simulink model "FunctionalArchitecture"  (R2022b)
settings: Solver=VariableStepAuto  StartTime=0.0  StopTime=10.0  RelTol=1e-3
undefined symbols (not defined in the file): Camera_data, Lidar, Posiont, Position, SpeedVacuum
settings Model: Creator=carol  LastModifiedBy=carol
settings OptimizationCC: ReuseModelBlockBuffer=on

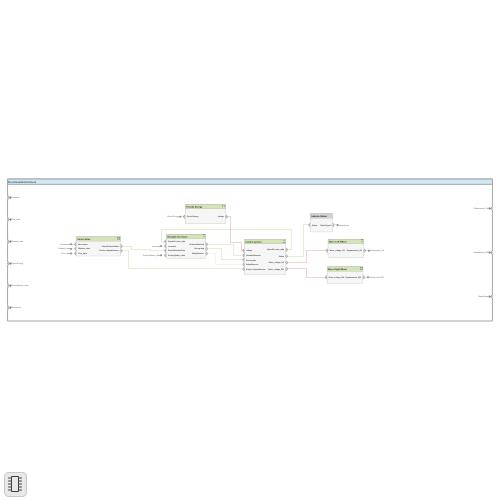
[thumbnail: Simulink's stored preview of the top-level diagram]
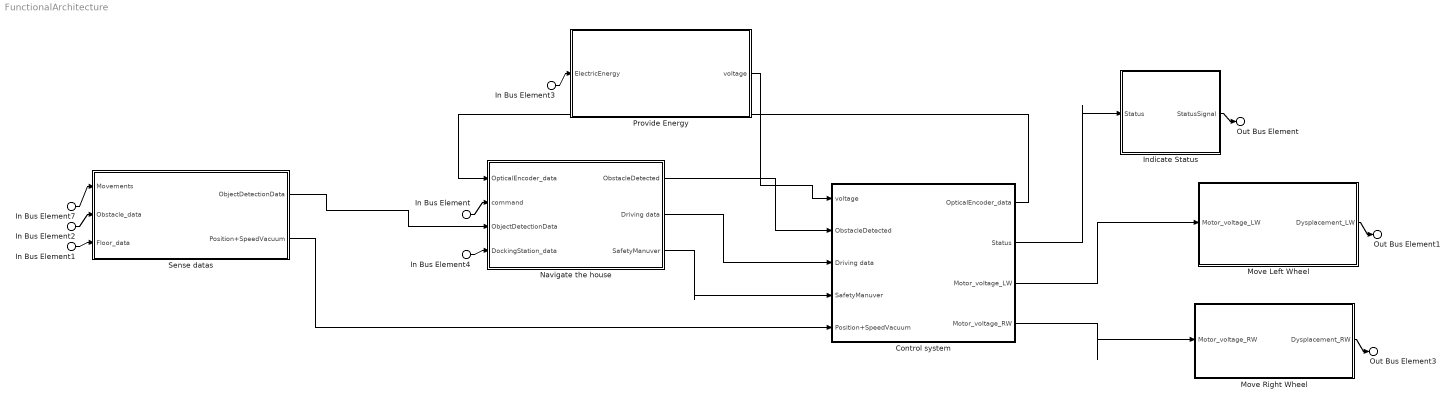
== system FunctionalArchitecture ==
  In Bus Element : Inport  PortName=command
  In Bus Element1 : Inport  Port=2  PortName=Floor_data
  In Bus Element2 : Inport  Port=3  PortName=Obstacle_data
  In Bus Element3 : Inport  Port=4  PortName=ElectricEnergy
  In Bus Element4 : Inport  Port=5  PortName=DockingStation_data
  In Bus Element7 : Inport  Port=6  PortName=Movements
  Control system : Subsystem
      settings: PortSchema="{\"entries\":[{\"content\":{\"headerSize\":26,\"margin\":15,\"minimumSpacing\":25,\"sides\":[{\"content\":{\"connectorIds\":[\"In1\",\"In2\",\"In4\",\"In3\",\"In5\"]},\"type\":\"ConnectorPlacement.EquallySpacedRectSide\",\"uuid\":\"6ae6270c-bff4-4a0d-8fba-8fdec87b0a05\"},{\"content\":{\"connectorIds\":[\"Out1\",\"Out2\",\"Out3\",\"Out4\"],\"side\":\"RIGHT\"},\"type\":\"ConnectorPlacement.EquallySpacedRectSide\",\"uuid\":\"f3a0045b-bb3b-40f9-afd5-e1537ff3eeca\"},{\"content\":{\"side\":\"TOP\"},\"type\":\"ConnectorPlacement.EquallySpacedRectSide\",\"uuid\":\"e89a58f2-90b0-468c-bb6a-95617af68e24\"}]},\"type\":\"ConnectorPlacement.EquallySpacedConnector\",\"uuid\":\"066eb43c-7b96-4660-9f29-628dd77a5b3b\"}],\"packageUris\":[\"http://schema.mathworks.com/mf0/Connector/R2020b\"],\"version\":\"1.0\"}"
  Indicate Status : Subsystem
      settings: PortSchema="{\"entries\":[{\"content\":{\"headerSize\":26,\"margin\":15,\"minimumSpacing\":25,\"sides\":[{\"content\":{\"connectorIds\":[\"In1\"]},\"type\":\"ConnectorPlacement.EquallySpacedRectSide\",\"uuid\":\"9cca9539-0a36-4124-b22c-ee31f3591a67\"},{\"content\":{\"connectorIds\":[\"Out1\"],\"side\":\"RIGHT\"},\"type\":\"ConnectorPlacement.EquallySpacedRectSide\",\"uuid\":\"eebe1ec1-c849-468b-8863-53f0cc841d23\"},{\"content\":{\"side\":\"TOP\"},\"type\":\"ConnectorPlacement.EquallySpacedRectSide\",\"uuid\":\"8f1c4dda-9d7f-4fb5-99d0-4e96ed432329\"}]},\"type\":\"ConnectorPlacement.EquallySpacedConnector\",\"uuid\":\"f7d57f3a-667c-4dfa-8f30-8433699dfbc6\"}],\"packageUris\":[\"http://schema.mathworks.com/mf0/Connector/R2020b\"],\"version\":\"1.0\"}"
  Move Left Wheel : Subsystem
      settings: PortSchema="{\"entries\":[{\"content\":{\"headerSize\":26,\"margin\":15,\"minimumSpacing\":25,\"sides\":[{\"content\":{\"connectorIds\":[\"In1\"]},\"type\":\"ConnectorPlacement.EquallySpacedRectSide\",\"uuid\":\"6ae6270c-bff4-4a0d-8fba-8fdec87b0a05\"},{\"content\":{\"connectorIds\":[\"Out1\"],\"side\":\"RIGHT\"},\"type\":\"ConnectorPlacement.EquallySpacedRectSide\",\"uuid\":\"f3a0045b-bb3b-40f9-afd5-e1537ff3eeca\"},{\"content\":{\"side\":\"TOP\"},\"type\":\"ConnectorPlacement.EquallySpacedRectSide\",\"uuid\":\"e89a58f2-90b0-468c-bb6a-95617af68e24\"}]},\"type\":\"ConnectorPlacement.EquallySpacedConnector\",\"uuid\":\"066eb43c-7b96-4660-9f29-628dd77a5b3b\"}],\"packageUris\":[\"http://schema.mathworks.com/mf0/Connector/R2020b\"],\"version\":\"1.0\"}"
  Move Right Wheel : Subsystem
      settings: PortSchema="{\"entries\":[{\"content\":{\"headerSize\":26,\"margin\":15,\"minimumSpacing\":25,\"sides\":[{\"content\":{\"connectorIds\":[\"In1\"]},\"type\":\"ConnectorPlacement.EquallySpacedRectSide\",\"uuid\":\"6ae6270c-bff4-4a0d-8fba-8fdec87b0a05\"},{\"content\":{\"connectorIds\":[\"Out1\"],\"side\":\"RIGHT\"},\"type\":\"ConnectorPlacement.EquallySpacedRectSide\",\"uuid\":\"f3a0045b-bb3b-40f9-afd5-e1537ff3eeca\"},{\"content\":{\"side\":\"TOP\"},\"type\":\"ConnectorPlacement.EquallySpacedRectSide\",\"uuid\":\"e89a58f2-90b0-468c-bb6a-95617af68e24\"}]},\"type\":\"ConnectorPlacement.EquallySpacedConnector\",\"uuid\":\"066eb43c-7b96-4660-9f29-628dd77a5b3b\"}],\"packageUris\":[\"http://schema.mathworks.com/mf0/Connector/R2020b\"],\"version\":\"1.0\"}"
  Navigate the house : Subsystem
      settings: PortSchema="{\"entries\":[{\"content\":{\"headerSize\":26,\"margin\":15,\"minimumSpacing\":25,\"sides\":[{\"content\":{\"connectorIds\":[\"In1\",\"In2\",\"In3\",\"In4\"]},\"type\":\"ConnectorPlacement.EquallySpacedRectSide\",\"uuid\":\"9cca9539-0a36-4124-b22c-ee31f3591a67\"},{\"content\":{\"connectorIds\":[\"Out1\",\"Out3\",\"Out2\"],\"side\":\"RIGHT\"},\"type\":\"ConnectorPlacement.EquallySpacedRectSide\",\"uuid\":\"eebe1ec1-c849-468b-8863-53f0cc841d23\"},{\"content\":{\"side\":\"TOP\"},\"type\":\"ConnectorPlacement.EquallySpacedRectSide\",\"uuid\":\"8f1c4dda-9d7f-4fb5-99d0-4e96ed432329\"}]},\"type\":\"ConnectorPlacement.EquallySpacedConnector\",\"uuid\":\"f7d57f3a-667c-4dfa-8f30-8433699dfbc6\"}],\"packageUris\":[\"http://schema.mathworks.com/mf0/Connector/R2020b\"],\"version\":\"1.0\"}"
  Provide Energy : Subsystem
      settings: PortSchema="{\"entries\":[{\"content\":{\"headerSize\":26,\"margin\":15,\"minimumSpacing\":25,\"sides\":[{\"content\":{\"connectorIds\":[\"In1\"]},\"type\":\"ConnectorPlacement.EquallySpacedRectSide\",\"uuid\":\"6ae6270c-bff4-4a0d-8fba-8fdec87b0a05\"},{\"content\":{\"connectorIds\":[\"Out1\"],\"side\":\"RIGHT\"},\"type\":\"ConnectorPlacement.EquallySpacedRectSide\",\"uuid\":\"f3a0045b-bb3b-40f9-afd5-e1537ff3eeca\"},{\"content\":{\"side\":\"TOP\"},\"type\":\"ConnectorPlacement.EquallySpacedRectSide\",\"uuid\":\"e89a58f2-90b0-468c-bb6a-95617af68e24\"}]},\"type\":\"ConnectorPlacement.EquallySpacedConnector\",\"uuid\":\"066eb43c-7b96-4660-9f29-628dd77a5b3b\"}],\"packageUris\":[\"http://schema.mathworks.com/mf0/Connector/R2020b\"],\"version\":\"1.0\"}"
  Sense datas : Subsystem
      settings: PortSchema="{\"entries\":[{\"content\":{\"headerSize\":26,\"margin\":15,\"minimumSpacing\":25,\"sides\":[{\"content\":{\"connectorIds\":[\"In1\",\"In2\",\"In3\"]},\"type\":\"ConnectorPlacement.EquallySpacedRectSide\",\"uuid\":\"6ae6270c-bff4-4a0d-8fba-8fdec87b0a05\"},{\"content\":{\"connectorIds\":[\"Out2\",\"Out1\"],\"side\":\"RIGHT\"},\"type\":\"ConnectorPlacement.EquallySpacedRectSide\",\"uuid\":\"f3a0045b-bb3b-40f9-afd5-e1537ff3eeca\"},{\"content\":{\"side\":\"TOP\"},\"type\":\"ConnectorPlacement.EquallySpacedRectSide\",\"uuid\":\"e89a58f2-90b0-468c-bb6a-95617af68e24\"}]},\"type\":\"ConnectorPlacement.EquallySpacedConnector\",\"uuid\":\"066eb43c-7b96-4660-9f29-628dd77a5b3b\"}],\"packageUris\":[\"http://schema.mathworks.com/mf0/Connector/R2020b\"],\"version\":\"1.0\"}"
  Out Bus Element1 : Outport  PortName=Displacement_LW
  Out Bus Element3 : Outport  Port=2  PortName=Displacement_RW
  Out Bus Element : Outport  Port=3  PortName=StatusSignal
  wires:
  Navigate the house/3(Driving data) -> Control system/4(Driving data)
  Provide Energy/1(voltage) -> Control system/1(voltage)
  In Bus Element3/1 -> Provide Energy/1(ElectricEnergy)
  Control system/3(Motor_voltage_LW) -> Move Left Wheel/1(Motor_voltage_LW)
  Control system/4(Motor_voltage_RW) -> Move Right Wheel/1(Motor_voltage_RW)
  Move Left Wheel/1(Dysplacement_LW) -> Out Bus Element1/1
  Move Right Wheel/1(Dysplacement_RW) -> Out Bus Element3/1
  In Bus Element7/1 -> Sense datas/1(Movements)
  In Bus Element2/1 -> Sense datas/2(Obstacle_data)
  In Bus Element1/1 -> Sense datas/3(Floor_data)
  Sense datas/2(ObjectDetectionData) -> Navigate the house/3(ObjectDetectionData)
  Sense datas/1(Position+SpeedVacuum) -> Control system/5(Position+SpeedVacuum)
  In Bus Element/1 -> Navigate the house/2(command)
  In Bus Element4/1 -> Navigate the house/4(DockingStation_data)
  Control system/1(OpticalEncoder_data) -> Navigate the house/1(OpticalEncoder_data)
  Indicate Status/1(StatusSignal) -> Out Bus Element/1
  Control system/2(Status) -> Indicate Status/1(Status)
  Navigate the house/1(ObstacleDetected) -> Control system/2(ObstacleDetected)
  Navigate the house/2(SafetyManuver) -> Control system/3(SafetyManuver)

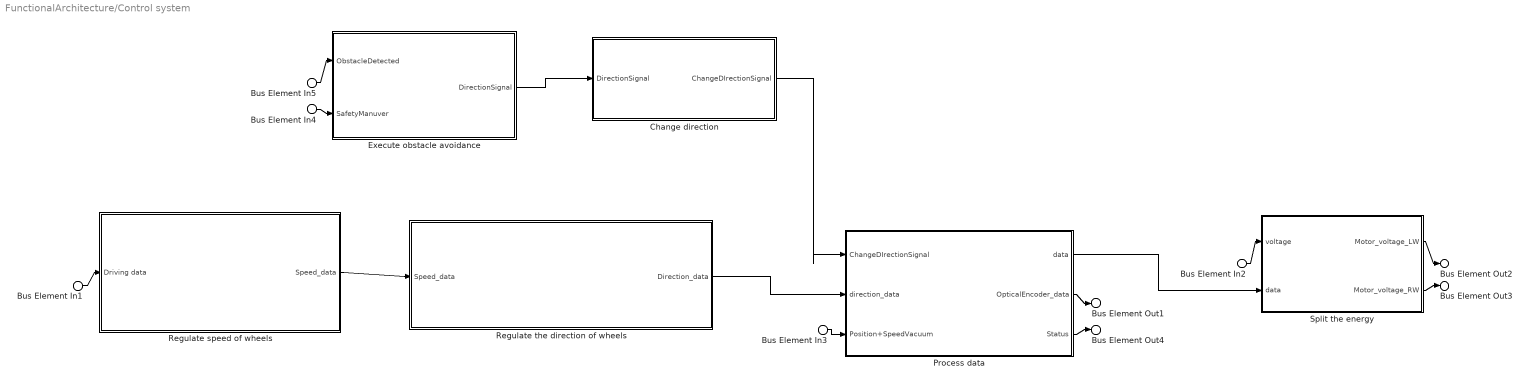
== system FunctionalArchitecture/Control system ==
  Bus Element In2 : Inport  PortName=voltage
  Bus Element In5 : Inport  Port=2  PortName=ObstacleDetected
  Bus Element In4 : Inport  Port=3  PortName=SafetyManuver
  Bus Element In1 : Inport  Port=4  PortName=Driving data
  Bus Element In3 : Inport  Port=5  PortName=Position+SpeedVacuum
  Change direction : Subsystem
      settings: PortSchema="{\"entries\":[{\"content\":{\"headerSize\":26,\"margin\":15,\"minimumSpacing\":25,\"sides\":[{\"content\":{\"connectorIds\":[\"In1\"]},\"type\":\"ConnectorPlacement.EquallySpacedRectSide\",\"uuid\":\"9cca9539-0a36-4124-b22c-ee31f3591a67\"},{\"content\":{\"connectorIds\":[\"Out1\"],\"side\":\"RIGHT\"},\"type\":\"ConnectorPlacement.EquallySpacedRectSide\",\"uuid\":\"eebe1ec1-c849-468b-8863-53f0cc841d23\"},{\"content\":{\"side\":\"TOP\"},\"type\":\"ConnectorPlacement.EquallySpacedRectSide\",\"uuid\":\"8f1c4dda-9d7f-4fb5-99d0-4e96ed432329\"}]},\"type\":\"ConnectorPlacement.EquallySpacedConnector\",\"uuid\":\"f7d57f3a-667c-4dfa-8f30-8433699dfbc6\"}],\"packageUris\":[\"http://schema.mathworks.com/mf0/Connector/R2020b\"],\"version\":\"1.0\"}"
  Execute obstacle avoidance : Subsystem
      settings: PortSchema="{\"entries\":[{\"content\":{\"headerSize\":26,\"margin\":15,\"minimumSpacing\":25,\"sides\":[{\"content\":{\"connectorIds\":[\"In1\",\"In2\"]},\"type\":\"ConnectorPlacement.EquallySpacedRectSide\",\"uuid\":\"9cca9539-0a36-4124-b22c-ee31f3591a67\"},{\"content\":{\"connectorIds\":[\"Out1\"],\"side\":\"RIGHT\"},\"type\":\"ConnectorPlacement.EquallySpacedRectSide\",\"uuid\":\"eebe1ec1-c849-468b-8863-53f0cc841d23\"},{\"content\":{\"side\":\"TOP\"},\"type\":\"ConnectorPlacement.EquallySpacedRectSide\",\"uuid\":\"8f1c4dda-9d7f-4fb5-99d0-4e96ed432329\"}]},\"type\":\"ConnectorPlacement.EquallySpacedConnector\",\"uuid\":\"f7d57f3a-667c-4dfa-8f30-8433699dfbc6\"}],\"packageUris\":[\"http://schema.mathworks.com/mf0/Connector/R2020b\"],\"version\":\"1.0\"}"
  Process data : Subsystem
      settings: PortSchema="{\"entries\":[{\"content\":{\"headerSize\":26,\"margin\":15,\"minimumSpacing\":25,\"sides\":[{\"content\":{\"connectorIds\":[\"In1\",\"In2\",\"In3\"]},\"type\":\"ConnectorPlacement.EquallySpacedRectSide\",\"uuid\":\"c0b5e0bb-d2bf-4d40-b1ad-0d63f5f2311e\"},{\"content\":{\"connectorIds\":[\"Out1\",\"Out2\",\"Out3\"],\"side\":\"RIGHT\"},\"type\":\"ConnectorPlacement.EquallySpacedRectSide\",\"uuid\":\"73104a81-7012-49ca-8030-68cbb7243dfa\"},{\"content\":{\"side\":\"TOP\"},\"type\":\"ConnectorPlacement.EquallySpacedRectSide\",\"uuid\":\"7c311739-eaa1-403c-a576-4458554363b2\"}]},\"type\":\"ConnectorPlacement.EquallySpacedConnector\",\"uuid\":\"83a80a93-0958-4176-98e5-b02d609066aa\"}],\"packageUris\":[\"http://schema.mathworks.com/mf0/Connector/R2020b\"],\"version\":\"1.0\"}"
  Regulate speed of wheels : Subsystem
      settings: PortSchema="{\"entries\":[{\"content\":{\"headerSize\":26,\"margin\":15,\"minimumSpacing\":25,\"sides\":[{\"content\":{\"connectorIds\":[\"In1\"]},\"type\":\"ConnectorPlacement.EquallySpacedRectSide\",\"uuid\":\"c0b5e0bb-d2bf-4d40-b1ad-0d63f5f2311e\"},{\"content\":{\"connectorIds\":[\"Out1\"],\"side\":\"RIGHT\"},\"type\":\"ConnectorPlacement.EquallySpacedRectSide\",\"uuid\":\"73104a81-7012-49ca-8030-68cbb7243dfa\"},{\"content\":{\"side\":\"TOP\"},\"type\":\"ConnectorPlacement.EquallySpacedRectSide\",\"uuid\":\"7c311739-eaa1-403c-a576-4458554363b2\"}]},\"type\":\"ConnectorPlacement.EquallySpacedConnector\",\"uuid\":\"83a80a93-0958-4176-98e5-b02d609066aa\"}],\"packageUris\":[\"http://schema.mathworks.com/mf0/Connector/R2020b\"],\"version\":\"1.0\"}"
  Regulate the direction of wheels : Subsystem
      settings: PortSchema="{\"entries\":[{\"content\":{\"headerSize\":26,\"margin\":15,\"minimumSpacing\":25,\"sides\":[{\"content\":{\"connectorIds\":[\"In1\"]},\"type\":\"ConnectorPlacement.EquallySpacedRectSide\",\"uuid\":\"c0b5e0bb-d2bf-4d40-b1ad-0d63f5f2311e\"},{\"content\":{\"connectorIds\":[\"Out1\"],\"side\":\"RIGHT\"},\"type\":\"ConnectorPlacement.EquallySpacedRectSide\",\"uuid\":\"73104a81-7012-49ca-8030-68cbb7243dfa\"},{\"content\":{\"side\":\"TOP\"},\"type\":\"ConnectorPlacement.EquallySpacedRectSide\",\"uuid\":\"7c311739-eaa1-403c-a576-4458554363b2\"}]},\"type\":\"ConnectorPlacement.EquallySpacedConnector\",\"uuid\":\"83a80a93-0958-4176-98e5-b02d609066aa\"}],\"packageUris\":[\"http://schema.mathworks.com/mf0/Connector/R2020b\"],\"version\":\"1.0\"}"
  Split the energy : Subsystem
      settings: PortSchema="{\"entries\":[{\"content\":{\"headerSize\":26,\"margin\":15,\"minimumSpacing\":25,\"sides\":[{\"content\":{\"connectorIds\":[\"In1\",\"In2\"]},\"type\":\"ConnectorPlacement.EquallySpacedRectSide\",\"uuid\":\"c0b5e0bb-d2bf-4d40-b1ad-0d63f5f2311e\"},{\"content\":{\"connectorIds\":[\"Out1\",\"Out2\"],\"side\":\"RIGHT\"},\"type\":\"ConnectorPlacement.EquallySpacedRectSide\",\"uuid\":\"73104a81-7012-49ca-8030-68cbb7243dfa\"},{\"content\":{\"side\":\"TOP\"},\"type\":\"ConnectorPlacement.EquallySpacedRectSide\",\"uuid\":\"7c311739-eaa1-403c-a576-4458554363b2\"}]},\"type\":\"ConnectorPlacement.EquallySpacedConnector\",\"uuid\":\"83a80a93-0958-4176-98e5-b02d609066aa\"}],\"packageUris\":[\"http://schema.mathworks.com/mf0/Connector/R2020b\"],\"version\":\"1.0\"}"
  Bus Element Out1 : Outport  PortName=OpticalEncoder_data
  Bus Element Out4 : Outport  Port=2  PortName=Status
  Bus Element Out2 : Outport  Port=3  PortName=Motor_voltage_LW
  Bus Element Out3 : Outport  Port=4  PortName=Motor_voltage_RW
  wires:
  Regulate speed of wheels/1(Speed_data) -> Regulate the direction of wheels/1(Speed_data)
  Split the energy/1(Motor_voltage_LW) -> Bus Element Out2/1
  Process data/1(data) -> Split the energy/2(data)
  Split the energy/2(Motor_voltage_RW) -> Bus Element Out3/1
  Regulate the direction of wheels/1(Direction_data) -> Process data/2(direction_data)
  Bus Element In1/1 -> Regulate speed of wheels/1(Driving data)
  Bus Element In3/1 -> Process data/3(Position+SpeedVacuum)
  Process data/2(OpticalEncoder_data) -> Bus Element Out1/1
  Bus Element In2/1 -> Split the energy/1(voltage)
  Execute obstacle avoidance/1(DirectionSignal) -> Change direction/1(DirectionSignal)
  Bus Element In5/1 -> Execute obstacle avoidance/1(ObstacleDetected)
  Change direction/1(ChangeDIrectionSignal) -> Process data/1(ChangeDIrectionSignal)
  Process data/3(Status) -> Bus Element Out4/1
  Bus Element In4/1 -> Execute obstacle avoidance/2(SafetyManuver)

== system FunctionalArchitecture/Indicate Status ==
  Bus Element In1 : Inport  PortName=Status
  Bus Element Out1 : Outport  PortName=StatusSignal

== system FunctionalArchitecture/Move Left Wheel ==
  Bus Element In1 : Inport  PortName=Motor_voltage_LW
  Bus Element Out1 : Outport  PortName=Dysplacement_LW

== system FunctionalArchitecture/Move Right Wheel ==
  Bus Element In1 : Inport  PortName=Motor_voltage_RW
  Bus Element Out1 : Outport  PortName=Dysplacement_RW

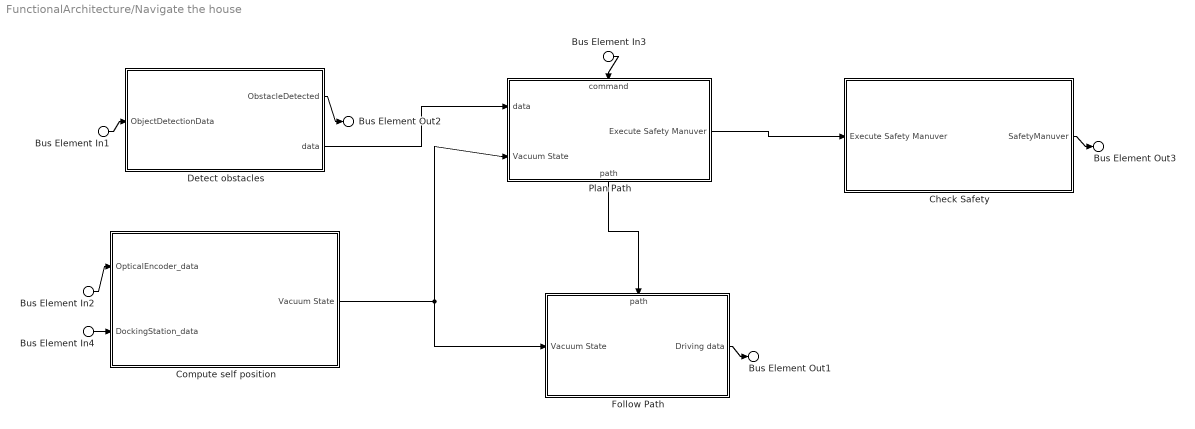
== system FunctionalArchitecture/Navigate the house ==
  Bus Element In2 : Inport  PortName=OpticalEncoder_data
  Bus Element In3 : Inport  Port=2  PortName=command
  Bus Element In1 : Inport  Port=3  PortName=ObjectDetectionData
  Bus Element In4 : Inport  Port=4  PortName=DockingStation_data
  Check Safety : Subsystem
      settings: PortSchema="{\"entries\":[{\"content\":{\"headerSize\":26,\"margin\":15,\"minimumSpacing\":25,\"sides\":[{\"content\":{\"connectorIds\":[\"In1\"]},\"type\":\"ConnectorPlacement.EquallySpacedRectSide\",\"uuid\":\"9cca9539-0a36-4124-b22c-ee31f3591a67\"},{\"content\":{\"connectorIds\":[\"Out1\"],\"side\":\"RIGHT\"},\"type\":\"ConnectorPlacement.EquallySpacedRectSide\",\"uuid\":\"eebe1ec1-c849-468b-8863-53f0cc841d23\"},{\"content\":{\"side\":\"TOP\"},\"type\":\"ConnectorPlacement.EquallySpacedRectSide\",\"uuid\":\"8f1c4dda-9d7f-4fb5-99d0-4e96ed432329\"}]},\"type\":\"ConnectorPlacement.EquallySpacedConnector\",\"uuid\":\"f7d57f3a-667c-4dfa-8f30-8433699dfbc6\"}],\"packageUris\":[\"http://schema.mathworks.com/mf0/Connector/R2020b\"],\"version\":\"1.0\"}"
  Compute self position : Subsystem
      settings: PortSchema="{\"entries\":[{\"content\":{\"headerSize\":26,\"margin\":15,\"minimumSpacing\":25,\"sides\":[{\"content\":{\"connectorIds\":[\"In1\",\"In2\"]},\"type\":\"ConnectorPlacement.EquallySpacedRectSide\",\"uuid\":\"9cca9539-0a36-4124-b22c-ee31f3591a67\"},{\"content\":{\"connectorIds\":[\"Out1\"],\"side\":\"RIGHT\"},\"type\":\"ConnectorPlacement.EquallySpacedRectSide\",\"uuid\":\"eebe1ec1-c849-468b-8863-53f0cc841d23\"},{\"content\":{\"side\":\"TOP\"},\"type\":\"ConnectorPlacement.EquallySpacedRectSide\",\"uuid\":\"8f1c4dda-9d7f-4fb5-99d0-4e96ed432329\"}]},\"type\":\"ConnectorPlacement.EquallySpacedConnector\",\"uuid\":\"f7d57f3a-667c-4dfa-8f30-8433699dfbc6\"}],\"packageUris\":[\"http://schema.mathworks.com/mf0/Connector/R2020b\"],\"version\":\"1.0\"}"
  "Detect obstacles " : Subsystem
      settings: PortSchema="{\"entries\":[{\"content\":{\"headerSize\":26,\"margin\":15,\"minimumSpacing\":25,\"sides\":[{\"content\":{\"connectorIds\":[\"In1\"]},\"type\":\"ConnectorPlacement.EquallySpacedRectSide\",\"uuid\":\"9cca9539-0a36-4124-b22c-ee31f3591a67\"},{\"content\":{\"connectorIds\":[\"Out1\",\"Out2\"],\"side\":\"RIGHT\"},\"type\":\"ConnectorPlacement.EquallySpacedRectSide\",\"uuid\":\"eebe1ec1-c849-468b-8863-53f0cc841d23\"},{\"content\":{\"side\":\"TOP\"},\"type\":\"ConnectorPlacement.EquallySpacedRectSide\",\"uuid\":\"8f1c4dda-9d7f-4fb5-99d0-4e96ed432329\"}]},\"type\":\"ConnectorPlacement.EquallySpacedConnector\",\"uuid\":\"f7d57f3a-667c-4dfa-8f30-8433699dfbc6\"}],\"packageUris\":[\"http://schema.mathworks.com/mf0/Connector/R2020b\"],\"version\":\"1.0\"}"
  Follow Path : Subsystem
      settings: PortSchema="{\"entries\":[{\"content\":{\"headerSize\":26,\"margin\":15,\"minimumSpacing\":25,\"sides\":[{\"content\":{\"connectorIds\":[\"In1\"]},\"type\":\"ConnectorPlacement.EquallySpacedRectSide\",\"uuid\":\"9cca9539-0a36-4124-b22c-ee31f3591a67\"},{\"content\":{\"connectorIds\":[\"Out1\"],\"side\":\"RIGHT\"},\"type\":\"ConnectorPlacement.EquallySpacedRectSide\",\"uuid\":\"eebe1ec1-c849-468b-8863-53f0cc841d23\"},{\"content\":{\"connectorIds\":[\"In2\"],\"side\":\"TOP\"},\"type\":\"ConnectorPlacement.EquallySpacedRectSide\",\"uuid\":\"8f1c4dda-9d7f-4fb5-99d0-4e96ed432329\"}]},\"type\":\"ConnectorPlacement.EquallySpacedConnector\",\"uuid\":\"f7d57f3a-667c-4dfa-8f30-8433699dfbc6\"}],\"packageUris\":[\"http://schema.mathworks.com/mf0/Connector/R2020b\"],\"version\":\"1.0\"}"
  Plan Path : Subsystem
      settings: PortSchema="{\"entries\":[{\"content\":{\"headerSize\":26,\"margin\":15,\"minimumSpacing\":25,\"sides\":[{\"content\":{\"connectorIds\":[\"In2\",\"In3\"]},\"type\":\"ConnectorPlacement.EquallySpacedRectSide\",\"uuid\":\"9cca9539-0a36-4124-b22c-ee31f3591a67\"},{\"content\":{\"connectorIds\":[\"Out2\"],\"side\":\"RIGHT\"},\"type\":\"ConnectorPlacement.EquallySpacedRectSide\",\"uuid\":\"eebe1ec1-c849-468b-8863-53f0cc841d23\"},{\"content\":{\"connectorIds\":[\"In1\"],\"side\":\"TOP\"},\"type\":\"ConnectorPlacement.EquallySpacedRectSide\",\"uuid\":\"8f1c4dda-9d7f-4fb5-99d0-4e96ed432329\"},{\"content\":{\"connectorIds\":[\"Out1\"],\"side\":\"BOTTOM\"},\"type\":\"ConnectorPlacement.EquallySpacedRectSide\",\"uuid\":\"2019f210-7520-495e-975e-724f2e2bbcde\"}]},\"type\":\"ConnectorPlacement.EquallySpacedConnector\",\"uuid\":\"f7d57f3a-667c-4dfa-8f30-8433699dfbc6\"}],\"packageUris\":[\"http://schema.mathworks.com/mf0/Connector/R2020b\"],\"version\":\"1.0\"}"
  Bus Element Out2 : Outport  PortName=ObstacleDetected
  Bus Element Out3 : Outport  Port=2  PortName=SafetyManuver
  Bus Element Out1 : Outport  Port=3  PortName=Driving data
  wires:
  Bus Element In1/1 -> "Detect obstacles "/1(ObjectDetectionData)
  "Detect obstacles "/2(data) -> Plan Path/2(data)
  Plan Path/2(Execute Safety Manuver) -> Check Safety/1(Execute Safety Manuver)
  Plan Path/1(path) -> Follow Path/2(path)
  Compute self position/1(Vacuum State) -> Follow Path/1(Vacuum State), Plan Path/3(Vacuum State)
  Follow Path/1(Driving data) -> Bus Element Out1/1
  Bus Element In3/1 -> Plan Path/1(command)
  Bus Element In4/1 -> Compute self position/2(DockingStation_data)
  Bus Element In2/1 -> Compute self position/1(OpticalEncoder_data)
  "Detect obstacles "/1(ObstacleDetected) -> Bus Element Out2/1
  Check Safety/1(SafetyManuver) -> Bus Element Out3/1

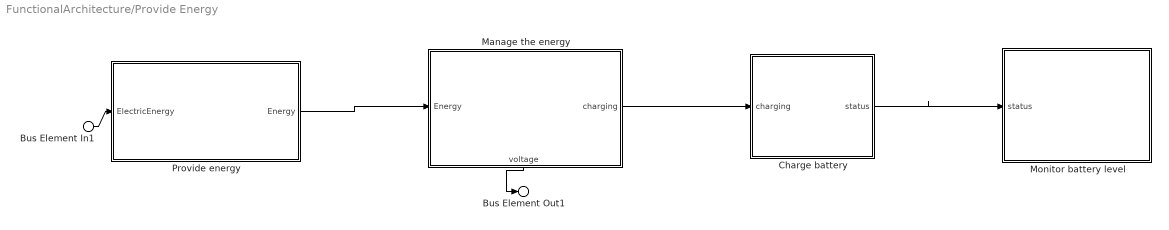
== system FunctionalArchitecture/Provide Energy ==
  Bus Element In1 : Inport  PortName=ElectricEnergy
  Charge battery : Subsystem
      settings: PortSchema="{\"entries\":[{\"content\":{\"headerSize\":26,\"margin\":15,\"minimumSpacing\":25,\"sides\":[{\"content\":{\"connectorIds\":[\"In1\"]},\"type\":\"ConnectorPlacement.EquallySpacedRectSide\",\"uuid\":\"9cca9539-0a36-4124-b22c-ee31f3591a67\"},{\"content\":{\"connectorIds\":[\"Out1\"],\"side\":\"RIGHT\"},\"type\":\"ConnectorPlacement.EquallySpacedRectSide\",\"uuid\":\"eebe1ec1-c849-468b-8863-53f0cc841d23\"},{\"content\":{\"side\":\"TOP\"},\"type\":\"ConnectorPlacement.EquallySpacedRectSide\",\"uuid\":\"8f1c4dda-9d7f-4fb5-99d0-4e96ed432329\"}]},\"type\":\"ConnectorPlacement.EquallySpacedConnector\",\"uuid\":\"f7d57f3a-667c-4dfa-8f30-8433699dfbc6\"}],\"packageUris\":[\"http://schema.mathworks.com/mf0/Connector/R2020b\"],\"version\":\"1.0\"}"
  Manage the energy : Subsystem
      settings: PortSchema="{\"entries\":[{\"content\":{\"headerSize\":26,\"margin\":15,\"minimumSpacing\":25,\"sides\":[{\"content\":{\"connectorIds\":[\"In1\"]},\"type\":\"ConnectorPlacement.EquallySpacedRectSide\",\"uuid\":\"c0b5e0bb-d2bf-4d40-b1ad-0d63f5f2311e\"},{\"content\":{\"connectorIds\":[\"Out2\"],\"side\":\"RIGHT\"},\"type\":\"ConnectorPlacement.EquallySpacedRectSide\",\"uuid\":\"73104a81-7012-49ca-8030-68cbb7243dfa\"},{\"content\":{\"side\":\"TOP\"},\"type\":\"ConnectorPlacement.EquallySpacedRectSide\",\"uuid\":\"7c311739-eaa1-403c-a576-4458554363b2\"},{\"content\":{\"connectorIds\":[\"Out1\"],\"side\":\"BOTTOM\"},\"type\":\"ConnectorPlacement.EquallySpacedRectSide\",\"uuid\":\"6353551f-44ff-4ee3-b4c3-711b036adab5\"}]},\"type\":\"ConnectorPlacement.EquallySpacedConnector\",\"uuid\":\"83a80a93-0958-4176-98e5-b02d609066aa\"}],\"packageUris\":[\"http://schema.mathworks.com/mf0/Connector/R2020b\"],\"version\":\"1.0\"}"
  Monitor battery level : Subsystem
      settings: PortSchema="{\"entries\":[{\"content\":{\"headerSize\":26,\"margin\":15,\"minimumSpacing\":25,\"sides\":[{\"content\":{\"connectorIds\":[\"In1\"]},\"type\":\"ConnectorPlacement.EquallySpacedRectSide\",\"uuid\":\"9cca9539-0a36-4124-b22c-ee31f3591a67\"},{\"content\":{\"side\":\"RIGHT\"},\"type\":\"ConnectorPlacement.EquallySpacedRectSide\",\"uuid\":\"eebe1ec1-c849-468b-8863-53f0cc841d23\"},{\"content\":{\"side\":\"TOP\"},\"type\":\"ConnectorPlacement.EquallySpacedRectSide\",\"uuid\":\"8f1c4dda-9d7f-4fb5-99d0-4e96ed432329\"}]},\"type\":\"ConnectorPlacement.EquallySpacedConnector\",\"uuid\":\"f7d57f3a-667c-4dfa-8f30-8433699dfbc6\"}],\"packageUris\":[\"http://schema.mathworks.com/mf0/Connector/R2020b\"],\"version\":\"1.0\"}"
  "Provide energy " : Subsystem
      settings: PortSchema="{\"entries\":[{\"content\":{\"headerSize\":26,\"margin\":15,\"minimumSpacing\":25,\"sides\":[{\"content\":{\"connectorIds\":[\"In1\"]},\"type\":\"ConnectorPlacement.EquallySpacedRectSide\",\"uuid\":\"9cca9539-0a36-4124-b22c-ee31f3591a67\"},{\"content\":{\"connectorIds\":[\"Out1\"],\"side\":\"RIGHT\"},\"type\":\"ConnectorPlacement.EquallySpacedRectSide\",\"uuid\":\"eebe1ec1-c849-468b-8863-53f0cc841d23\"},{\"content\":{\"side\":\"TOP\"},\"type\":\"ConnectorPlacement.EquallySpacedRectSide\",\"uuid\":\"8f1c4dda-9d7f-4fb5-99d0-4e96ed432329\"}]},\"type\":\"ConnectorPlacement.EquallySpacedConnector\",\"uuid\":\"f7d57f3a-667c-4dfa-8f30-8433699dfbc6\"}],\"packageUris\":[\"http://schema.mathworks.com/mf0/Connector/R2020b\"],\"version\":\"1.0\"}"
  Bus Element Out1 : Outport  PortName=voltage
  wires:
  Bus Element In1/1 -> "Provide energy "/1(ElectricEnergy)
  "Provide energy "/1(Energy) -> Manage the energy/1(Energy)
  Manage the energy/2(charging) -> Charge battery/1(charging)
  Charge battery/1(status) -> Monitor battery level/1(status)
  Manage the energy/1(voltage) -> Bus Element Out1/1

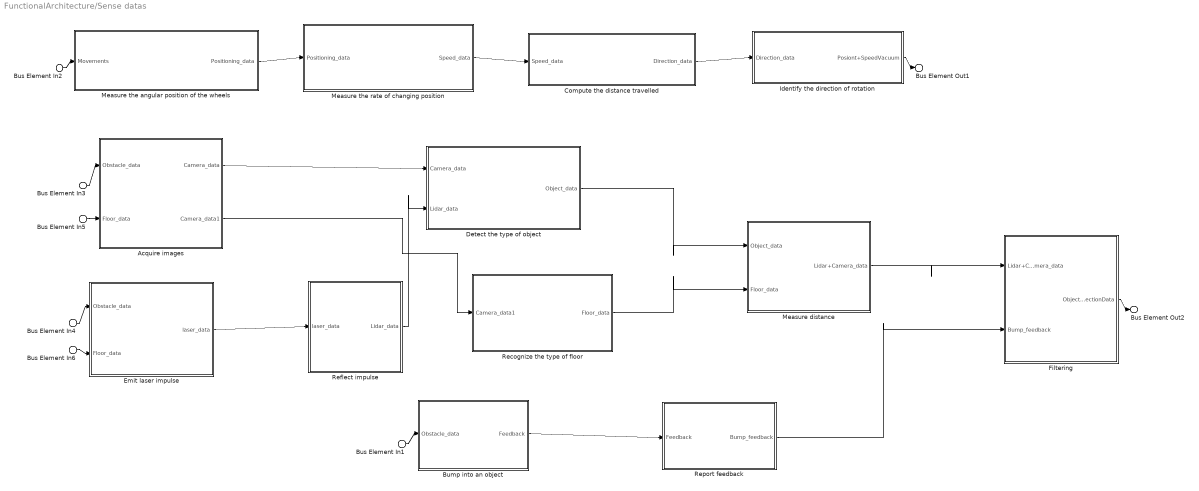
== system FunctionalArchitecture/Sense datas ==
  Bus Element In2 : Inport  PortName=Movements
  Bus Element In3 : Inport  Port=2  PortName=Obstacle_data
  Bus Element In4 : Inport  Port=2  PortName=Obstacle_data
  Bus Element In1 : Inport  Port=2  PortName=Obstacle_data
  Bus Element In5 : Inport  Port=3  PortName=Floor_data
  Bus Element In6 : Inport  Port=3  PortName=Floor_data
  Acquire images : Subsystem
      settings: PortSchema="{\"entries\":[{\"content\":{\"headerSize\":26,\"margin\":15,\"minimumSpacing\":25,\"sides\":[{\"content\":{\"connectorIds\":[\"In1\",\"In2\"]},\"type\":\"ConnectorPlacement.EquallySpacedRectSide\",\"uuid\":\"c0b5e0bb-d2bf-4d40-b1ad-0d63f5f2311e\"},{\"content\":{\"connectorIds\":[\"Out1\",\"Out2\"],\"side\":\"RIGHT\"},\"type\":\"ConnectorPlacement.EquallySpacedRectSide\",\"uuid\":\"73104a81-7012-49ca-8030-68cbb7243dfa\"},{\"content\":{\"side\":\"TOP\"},\"type\":\"ConnectorPlacement.EquallySpacedRectSide\",\"uuid\":\"7c311739-eaa1-403c-a576-4458554363b2\"}]},\"type\":\"ConnectorPlacement.EquallySpacedConnector\",\"uuid\":\"83a80a93-0958-4176-98e5-b02d609066aa\"}],\"packageUris\":[\"http://schema.mathworks.com/mf0/Connector/R2020b\"],\"version\":\"1.0\"}"
  Bump into an object : Subsystem
      settings: PortSchema="{\"entries\":[{\"content\":{\"headerSize\":26,\"margin\":15,\"minimumSpacing\":25,\"sides\":[{\"content\":{\"connectorIds\":[\"In1\"]},\"type\":\"ConnectorPlacement.EquallySpacedRectSide\",\"uuid\":\"9cca9539-0a36-4124-b22c-ee31f3591a67\"},{\"content\":{\"connectorIds\":[\"Out1\"],\"side\":\"RIGHT\"},\"type\":\"ConnectorPlacement.EquallySpacedRectSide\",\"uuid\":\"eebe1ec1-c849-468b-8863-53f0cc841d23\"},{\"content\":{\"side\":\"TOP\"},\"type\":\"ConnectorPlacement.EquallySpacedRectSide\",\"uuid\":\"8f1c4dda-9d7f-4fb5-99d0-4e96ed432329\"}]},\"type\":\"ConnectorPlacement.EquallySpacedConnector\",\"uuid\":\"f7d57f3a-667c-4dfa-8f30-8433699dfbc6\"}],\"packageUris\":[\"http://schema.mathworks.com/mf0/Connector/R2020b\"],\"version\":\"1.0\"}"
  "Compute the distance travelled " : Subsystem
      settings: PortSchema="{\"entries\":[{\"content\":{\"headerSize\":26,\"margin\":15,\"minimumSpacing\":25,\"sides\":[{\"content\":{\"connectorIds\":[\"In1\"]},\"type\":\"ConnectorPlacement.EquallySpacedRectSide\",\"uuid\":\"9cca9539-0a36-4124-b22c-ee31f3591a67\"},{\"content\":{\"connectorIds\":[\"Out1\"],\"side\":\"RIGHT\"},\"type\":\"ConnectorPlacement.EquallySpacedRectSide\",\"uuid\":\"eebe1ec1-c849-468b-8863-53f0cc841d23\"},{\"content\":{\"side\":\"TOP\"},\"type\":\"ConnectorPlacement.EquallySpacedRectSide\",\"uuid\":\"8f1c4dda-9d7f-4fb5-99d0-4e96ed432329\"}]},\"type\":\"ConnectorPlacement.EquallySpacedConnector\",\"uuid\":\"f7d57f3a-667c-4dfa-8f30-8433699dfbc6\"}],\"packageUris\":[\"http://schema.mathworks.com/mf0/Connector/R2020b\"],\"version\":\"1.0\"}"
  Detect the type of object : Subsystem
      settings: PortSchema="{\"entries\":[{\"content\":{\"headerSize\":26,\"margin\":15,\"minimumSpacing\":25,\"sides\":[{\"content\":{\"connectorIds\":[\"In1\",\"In2\"]},\"type\":\"ConnectorPlacement.EquallySpacedRectSide\",\"uuid\":\"c0b5e0bb-d2bf-4d40-b1ad-0d63f5f2311e\"},{\"content\":{\"connectorIds\":[\"Out1\"],\"side\":\"RIGHT\"},\"type\":\"ConnectorPlacement.EquallySpacedRectSide\",\"uuid\":\"73104a81-7012-49ca-8030-68cbb7243dfa\"},{\"content\":{\"side\":\"TOP\"},\"type\":\"ConnectorPlacement.EquallySpacedRectSide\",\"uuid\":\"7c311739-eaa1-403c-a576-4458554363b2\"}]},\"type\":\"ConnectorPlacement.EquallySpacedConnector\",\"uuid\":\"83a80a93-0958-4176-98e5-b02d609066aa\"}],\"packageUris\":[\"http://schema.mathworks.com/mf0/Connector/R2020b\"],\"version\":\"1.0\"}"
  Emit laser impulse : Subsystem
      settings: PortSchema="{\"entries\":[{\"content\":{\"headerSize\":26,\"margin\":15,\"minimumSpacing\":25,\"sides\":[{\"content\":{\"connectorIds\":[\"In2\",\"In1\"]},\"type\":\"ConnectorPlacement.EquallySpacedRectSide\",\"uuid\":\"c0b5e0bb-d2bf-4d40-b1ad-0d63f5f2311e\"},{\"content\":{\"connectorIds\":[\"Out1\"],\"side\":\"RIGHT\"},\"type\":\"ConnectorPlacement.EquallySpacedRectSide\",\"uuid\":\"73104a81-7012-49ca-8030-68cbb7243dfa\"},{\"content\":{\"side\":\"TOP\"},\"type\":\"ConnectorPlacement.EquallySpacedRectSide\",\"uuid\":\"7c311739-eaa1-403c-a576-4458554363b2\"},{\"content\":{\"side\":\"BOTTOM\"},\"type\":\"ConnectorPlacement.EquallySpacedRectSide\",\"uuid\":\"1fdf15b1-8a8d-4350-bda7-0c86e31633d1\"}]},\"type\":\"ConnectorPlacement.EquallySpacedConnector\",\"uuid\":\"83a80a93-0958-4176-98e5-b02d609066aa\"}],\"packageUris\":[\"http://schema.mathworks.com/mf0/Connector/R2020b\"],\"version\":\"1.0\"}"
  Filtering : Subsystem
      settings: PortSchema="{\"entries\":[{\"content\":{\"headerSize\":26,\"margin\":15,\"minimumSpacing\":25,\"sides\":[{\"content\":{\"connectorIds\":[\"In1\",\"In2\"]},\"type\":\"ConnectorPlacement.EquallySpacedRectSide\",\"uuid\":\"9cca9539-0a36-4124-b22c-ee31f3591a67\"},{\"content\":{\"connectorIds\":[\"Out1\"],\"side\":\"RIGHT\"},\"type\":\"ConnectorPlacement.EquallySpacedRectSide\",\"uuid\":\"eebe1ec1-c849-468b-8863-53f0cc841d23\"},{\"content\":{\"side\":\"TOP\"},\"type\":\"ConnectorPlacement.EquallySpacedRectSide\",\"uuid\":\"8f1c4dda-9d7f-4fb5-99d0-4e96ed432329\"}]},\"type\":\"ConnectorPlacement.EquallySpacedConnector\",\"uuid\":\"f7d57f3a-667c-4dfa-8f30-8433699dfbc6\"}],\"packageUris\":[\"http://schema.mathworks.com/mf0/Connector/R2020b\"],\"version\":\"1.0\"}"
  "Identify the direction of rotation " : Subsystem
      settings: PortSchema="{\"entries\":[{\"content\":{\"headerSize\":26,\"margin\":15,\"minimumSpacing\":25,\"sides\":[{\"content\":{\"connectorIds\":[\"In1\"]},\"type\":\"ConnectorPlacement.EquallySpacedRectSide\",\"uuid\":\"9cca9539-0a36-4124-b22c-ee31f3591a67\"},{\"content\":{\"connectorIds\":[\"Out1\"],\"side\":\"RIGHT\"},\"type\":\"ConnectorPlacement.EquallySpacedRectSide\",\"uuid\":\"eebe1ec1-c849-468b-8863-53f0cc841d23\"},{\"content\":{\"side\":\"TOP\"},\"type\":\"ConnectorPlacement.EquallySpacedRectSide\",\"uuid\":\"8f1c4dda-9d7f-4fb5-99d0-4e96ed432329\"}]},\"type\":\"ConnectorPlacement.EquallySpacedConnector\",\"uuid\":\"f7d57f3a-667c-4dfa-8f30-8433699dfbc6\"}],\"packageUris\":[\"http://schema.mathworks.com/mf0/Connector/R2020b\"],\"version\":\"1.0\"}"
  Measure distance : Subsystem
      settings: PortSchema="{\"entries\":[{\"content\":{\"headerSize\":26,\"margin\":15,\"minimumSpacing\":25,\"sides\":[{\"content\":{\"connectorIds\":[\"In1\",\"In2\"]},\"type\":\"ConnectorPlacement.EquallySpacedRectSide\",\"uuid\":\"c0b5e0bb-d2bf-4d40-b1ad-0d63f5f2311e\"},{\"content\":{\"connectorIds\":[\"Out1\"],\"side\":\"RIGHT\"},\"type\":\"ConnectorPlacement.EquallySpacedRectSide\",\"uuid\":\"73104a81-7012-49ca-8030-68cbb7243dfa\"},{\"content\":{\"side\":\"TOP\"},\"type\":\"ConnectorPlacement.EquallySpacedRectSide\",\"uuid\":\"7c311739-eaa1-403c-a576-4458554363b2\"}]},\"type\":\"ConnectorPlacement.EquallySpacedConnector\",\"uuid\":\"83a80a93-0958-4176-98e5-b02d609066aa\"}],\"packageUris\":[\"http://schema.mathworks.com/mf0/Connector/R2020b\"],\"version\":\"1.0\"}"
  Measure the angular position of the wheels : Subsystem
      settings: PortSchema="{\"entries\":[{\"content\":{\"headerSize\":26,\"margin\":15,\"minimumSpacing\":25,\"sides\":[{\"content\":{\"connectorIds\":[\"In1\"]},\"type\":\"ConnectorPlacement.EquallySpacedRectSide\",\"uuid\":\"9cca9539-0a36-4124-b22c-ee31f3591a67\"},{\"content\":{\"connectorIds\":[\"Out1\"],\"side\":\"RIGHT\"},\"type\":\"ConnectorPlacement.EquallySpacedRectSide\",\"uuid\":\"eebe1ec1-c849-468b-8863-53f0cc841d23\"},{\"content\":{\"side\":\"TOP\"},\"type\":\"ConnectorPlacement.EquallySpacedRectSide\",\"uuid\":\"8f1c4dda-9d7f-4fb5-99d0-4e96ed432329\"}]},\"type\":\"ConnectorPlacement.EquallySpacedConnector\",\"uuid\":\"f7d57f3a-667c-4dfa-8f30-8433699dfbc6\"}],\"packageUris\":[\"http://schema.mathworks.com/mf0/Connector/R2020b\"],\"version\":\"1.0\"}"
  Measure the rate of changing position : Subsystem
      settings: PortSchema="{\"entries\":[{\"content\":{\"headerSize\":26,\"margin\":15,\"minimumSpacing\":25,\"sides\":[{\"content\":{\"connectorIds\":[\"In1\"]},\"type\":\"ConnectorPlacement.EquallySpacedRectSide\",\"uuid\":\"9cca9539-0a36-4124-b22c-ee31f3591a67\"},{\"content\":{\"connectorIds\":[\"Out1\"],\"side\":\"RIGHT\"},\"type\":\"ConnectorPlacement.EquallySpacedRectSide\",\"uuid\":\"eebe1ec1-c849-468b-8863-53f0cc841d23\"},{\"content\":{\"side\":\"TOP\"},\"type\":\"ConnectorPlacement.EquallySpacedRectSide\",\"uuid\":\"8f1c4dda-9d7f-4fb5-99d0-4e96ed432329\"}]},\"type\":\"ConnectorPlacement.EquallySpacedConnector\",\"uuid\":\"f7d57f3a-667c-4dfa-8f30-8433699dfbc6\"}],\"packageUris\":[\"http://schema.mathworks.com/mf0/Connector/R2020b\"],\"version\":\"1.0\"}"
  Recognize the type of floor : Subsystem
      settings: PortSchema="{\"entries\":[{\"content\":{\"headerSize\":26,\"margin\":15,\"minimumSpacing\":25,\"sides\":[{\"content\":{\"connectorIds\":[\"In1\"]},\"type\":\"ConnectorPlacement.EquallySpacedRectSide\",\"uuid\":\"c0b5e0bb-d2bf-4d40-b1ad-0d63f5f2311e\"},{\"content\":{\"connectorIds\":[\"Out1\"],\"side\":\"RIGHT\"},\"type\":\"ConnectorPlacement.EquallySpacedRectSide\",\"uuid\":\"73104a81-7012-49ca-8030-68cbb7243dfa\"},{\"content\":{\"side\":\"TOP\"},\"type\":\"ConnectorPlacement.EquallySpacedRectSide\",\"uuid\":\"7c311739-eaa1-403c-a576-4458554363b2\"}]},\"type\":\"ConnectorPlacement.EquallySpacedConnector\",\"uuid\":\"83a80a93-0958-4176-98e5-b02d609066aa\"}],\"packageUris\":[\"http://schema.mathworks.com/mf0/Connector/R2020b\"],\"version\":\"1.0\"}"
  Reflect impulse : Subsystem
      settings: PortSchema="{\"entries\":[{\"content\":{\"headerSize\":26,\"margin\":15,\"minimumSpacing\":25,\"sides\":[{\"content\":{\"connectorIds\":[\"In1\"]},\"type\":\"ConnectorPlacement.EquallySpacedRectSide\",\"uuid\":\"c0b5e0bb-d2bf-4d40-b1ad-0d63f5f2311e\"},{\"content\":{\"connectorIds\":[\"Out1\"],\"side\":\"RIGHT\"},\"type\":\"ConnectorPlacement.EquallySpacedRectSide\",\"uuid\":\"73104a81-7012-49ca-8030-68cbb7243dfa\"},{\"content\":{\"side\":\"TOP\"},\"type\":\"ConnectorPlacement.EquallySpacedRectSide\",\"uuid\":\"7c311739-eaa1-403c-a576-4458554363b2\"}]},\"type\":\"ConnectorPlacement.EquallySpacedConnector\",\"uuid\":\"83a80a93-0958-4176-98e5-b02d609066aa\"}],\"packageUris\":[\"http://schema.mathworks.com/mf0/Connector/R2020b\"],\"version\":\"1.0\"}"
  Report feedback : Subsystem
      settings: PortSchema="{\"entries\":[{\"content\":{\"headerSize\":26,\"margin\":15,\"minimumSpacing\":25,\"sides\":[{\"content\":{\"connectorIds\":[\"In1\"]},\"type\":\"ConnectorPlacement.EquallySpacedRectSide\",\"uuid\":\"9cca9539-0a36-4124-b22c-ee31f3591a67\"},{\"content\":{\"connectorIds\":[\"Out1\"],\"side\":\"RIGHT\"},\"type\":\"ConnectorPlacement.EquallySpacedRectSide\",\"uuid\":\"eebe1ec1-c849-468b-8863-53f0cc841d23\"},{\"content\":{\"side\":\"TOP\"},\"type\":\"ConnectorPlacement.EquallySpacedRectSide\",\"uuid\":\"8f1c4dda-9d7f-4fb5-99d0-4e96ed432329\"}]},\"type\":\"ConnectorPlacement.EquallySpacedConnector\",\"uuid\":\"f7d57f3a-667c-4dfa-8f30-8433699dfbc6\"}],\"packageUris\":[\"http://schema.mathworks.com/mf0/Connector/R2020b\"],\"version\":\"1.0\"}"
  Bus Element Out1 : Outport  PortName=Position+SpeedVacuum
  Bus Element Out2 : Outport  Port=2  PortName=ObjectDetectionData
  wires:
  Bus Element In6/1 -> Emit laser impulse/1(Floor_data)
  Recognize the type of floor/1(Floor_data) -> Measure distance/2(Floor_data)
  Emit laser impulse/1(laser_data) -> Reflect impulse/1(laser_data)
  Bus Element In4/1 -> Emit laser impulse/2(Obstacle_data)
  Acquire images/1(Camera_data) -> Detect the type of object/1(Camera_data)
  Detect the type of object/1(Object_data) -> Measure distance/1(Object_data)
  Reflect impulse/1(Lidar_data) -> Detect the type of object/2(Lidar_data)
  Bus Element In5/1 -> Acquire images/2(Floor_data)
  Bus Element In3/1 -> Acquire images/1(Obstacle_data)
  Acquire images/2(Camera_data1) -> Recognize the type of floor/1(Camera_data1)
  Bus Element In2/1 -> Measure the angular position of the wheels/1(Movements)
  Measure the angular position of the wheels/1(Positioning_data) -> Measure the rate of changing position/1(Positioning_data)
  Measure the rate of changing position/1(Speed_data) -> "Compute the distance travelled "/1(Speed_data)
  "Compute the distance travelled "/1(Direction_data) -> "Identify the direction of rotation "/1(Direction_data)
  "Identify the direction of rotation "/1(Posiont+SpeedVacuum) -> Bus Element Out1/1
  Bus Element In1/1 -> Bump into an object/1(Obstacle_data)
  Bump into an object/1(Feedback) -> Report feedback/1(Feedback)
  Report feedback/1(Bump_feedback) -> Filtering/2(Bump_feedback)
  Measure distance/1(Lidar+Camera_data) -> Filtering/1(Lidar+Camera_data)
  Filtering/1(ObjectDetectionData) -> Bus Element Out2/1

== system FunctionalArchitecture/Control system/Change direction ==
  Bus Element In1 : Inport  PortName=DirectionSignal
  Bus Element Out1 : Outport  PortName=ChangeDIrectionSignal

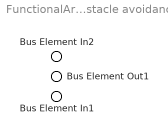
== system FunctionalArchitecture/Control system/Execute obstacle avoidance ==
  Bus Element In2 : Inport  PortName=ObstacleDetected
  Bus Element In1 : Inport  Port=2  PortName=SafetyManuver
  Bus Element Out1 : Outport  PortName=DirectionSignal

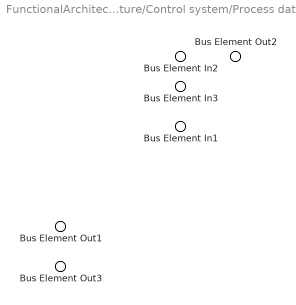
== system FunctionalArchitecture/Control system/Process data ==
  Bus Element In3 : Inport  PortName=ChangeDIrectionSignal
  Bus Element In2 : Inport  Port=2  PortName=direction_data
  Bus Element In1 : Inport  Port=3  PortName=Position+SpeedVacuum
  Bus Element Out2 : Outport  PortName=data
  Bus Element Out1 : Outport  Port=2  PortName=OpticalEncoder_data
  Bus Element Out3 : Outport  Port=3  PortName=Status

== system FunctionalArchitecture/Control system/Regulate speed of wheels ==
  Bus Element In1 : Inport  PortName=Driving data
  Bus Element Out1 : Outport  PortName=Speed_data

== system FunctionalArchitecture/Control system/Regulate the direction of wheels ==
  Bus Element In1 : Inport  PortName=Speed_data
  Bus Element Out1 : Outport  PortName=Direction_data

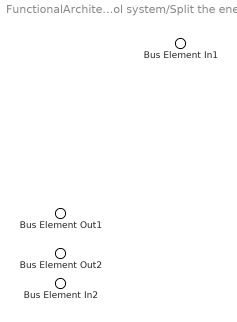
== system FunctionalArchitecture/Control system/Split the energy ==
  Bus Element In1 : Inport  PortName=voltage
  Bus Element In2 : Inport  Port=2  PortName=data
  Bus Element Out1 : Outport  PortName=Motor_voltage_LW
  Bus Element Out2 : Outport  Port=2  PortName=Motor_voltage_RW

== system FunctionalArchitecture/Navigate the house/Check Safety ==
  Bus Element In1 : Inport  PortName=Execute Safety Manuver
  Bus Element Out1 : Outport  PortName=SafetyManuver

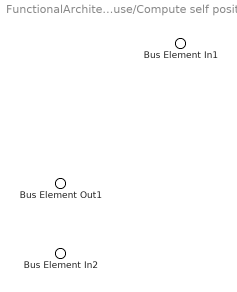
== system FunctionalArchitecture/Navigate the house/Compute self position ==
  Bus Element In1 : Inport  PortName=OpticalEncoder_data
  Bus Element In2 : Inport  Port=2  PortName=DockingStation_data
  Bus Element Out1 : Outport  PortName=Vacuum State

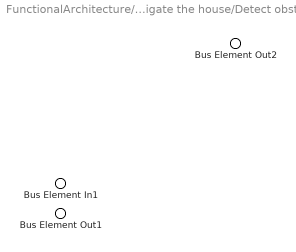
== system FunctionalArchitecture/Navigate the house/Detect obstacles  ==
  Bus Element In1 : Inport  PortName=ObjectDetectionData
  Bus Element Out2 : Outport  PortName=ObstacleDetected
  Bus Element Out1 : Outport  Port=2  PortName=data

== system FunctionalArchitecture/Navigate the house/Follow Path ==
  Bus Element In2 : Inport  PortName=Vacuum State
  Bus Element In1 : Inport  Port=2  PortName=path
  Bus Element Out1 : Outport  PortName=Driving data

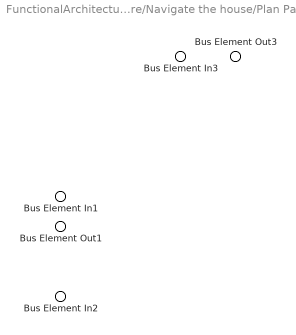
== system FunctionalArchitecture/Navigate the house/Plan Path ==
  Bus Element In3 : Inport  PortName=command
  Bus Element In1 : Inport  Port=2  PortName=data
  Bus Element In2 : Inport  Port=3  PortName=Vacuum State
  Bus Element Out3 : Outport  PortName=path
  Bus Element Out1 : Outport  Port=2  PortName=Execute Safety Manuver

== system FunctionalArchitecture/Provide Energy/Charge battery ==
  Bus Element In1 : Inport  PortName=charging
  Bus Element Out1 : Outport  PortName=status

== system FunctionalArchitecture/Provide Energy/Manage the energy ==
  Bus Element In1 : Inport  PortName=Energy
  Bus Element Out2 : Outport  PortName=voltage
  Bus Element Out1 : Outport  Port=2  PortName=charging

== system FunctionalArchitecture/Provide Energy/Monitor battery level ==
  Bus Element In1 : Inport  PortName=status

== system FunctionalArchitecture/Provide Energy/Provide energy  ==
  Bus Element In1 : Inport  PortName=ElectricEnergy
  Bus Element Out1 : Outport  PortName=Energy

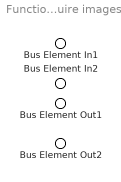
== system FunctionalArchitecture/Sense datas/Acquire images ==
  Bus Element In1 : Inport  PortName=Obstacle_data
  Bus Element In2 : Inport  Port=2  PortName=Floor_data
  Bus Element Out1 : Outport  PortName=Camera_data
  Bus Element Out2 : Outport  Port=2  PortName=Camera_data1

== system FunctionalArchitecture/Sense datas/Bump into an object ==
  Bus Element In1 : Inport  PortName=Obstacle_data
  Bus Element Out1 : Outport  PortName=Feedback

== system FunctionalArchitecture/Sense datas/Compute the distance travelled  ==
  Bus Element In1 : Inport  PortName=Speed_data
  Bus Element Out1 : Outport  PortName=Direction_data

== system FunctionalArchitecture/Sense datas/Detect the type of object ==
  Bus Element In1 : Inport  PortName=Camera_data
  Bus Element In2 : Inport  Port=2  PortName=Lidar_data
  Bus Element Out1 : Outport  PortName=Object_data

== system FunctionalArchitecture/Sense datas/Emit laser impulse ==
  Bus Element In2 : Inport  PortName=Floor_data
  Bus Element In1 : Inport  Port=2  PortName=Obstacle_data
  Bus Element Out1 : Outport  PortName=laser_data

== system FunctionalArchitecture/Sense datas/Filtering ==
  Bus Element In2 : Inport  PortName=Lidar+Camera_data
  Bus Element In1 : Inport  Port=2  PortName=Bump_feedback
  Bus Element Out1 : Outport  PortName=ObjectDetectionData

== system FunctionalArchitecture/Sense datas/Identify the direction of rotation  ==
  Bus Element In1 : Inport  PortName=Direction_data
  Bus Element Out1 : Outport  PortName=Posiont+SpeedVacuum

== system FunctionalArchitecture/Sense datas/Measure distance ==
  Bus Element In1 : Inport  PortName=Object_data
  Bus Element In2 : Inport  Port=2  PortName=Floor_data
  Bus Element Out1 : Outport  PortName=Lidar+Camera_data

== system FunctionalArchitecture/Sense datas/Measure the angular position of the wheels ==
  Bus Element In1 : Inport  PortName=Movements
  Bus Element Out1 : Outport  PortName=Positioning_data

== system FunctionalArchitecture/Sense datas/Measure the rate of changing position ==
  Bus Element In1 : Inport  PortName=Positioning_data
  Bus Element Out1 : Outport  PortName=Speed_data

== system FunctionalArchitecture/Sense datas/Recognize the type of floor ==
  Bus Element In1 : Inport  PortName=Camera_data1
  Bus Element Out1 : Outport  PortName=Floor_data

== system FunctionalArchitecture/Sense datas/Reflect impulse ==
  Bus Element In1 : Inport  PortName=laser_data
  Bus Element Out2 : Outport  PortName=Lidar_data

== system FunctionalArchitecture/Sense datas/Report feedback ==
  Bus Element In1 : Inport  PortName=Feedback
  Bus Element Out1 : Outport  PortName=Bump_feedback
